simulink model "SmithPredictor"  (R2014a)
settings: Solver=ode45  StartTime=0.0  StopTime=200  RelTol=1e-3
libraries: simulink x2
settings Model: Creator=tri  LastModifiedBy=tri

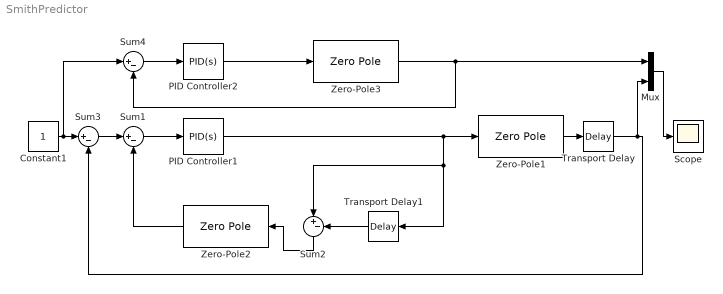
== system SmithPredictor ==
  Constant1 : Constant
  Mux : Mux  Inputs=2
  PID Controller1 : simulink/Continuous/PID Controller  Controller=PID  TimeDomain=Continuous-time  SampleTime=1  IntegratorMethod=Forward Euler  FilterMethod=Forward Euler  Form=Parallel  P=3  I=1/50  D=0  N=500  InitialConditionSource=internal  InitialConditionForIntegrator=0  InitialConditionForFilter=0  ExternalReset=none  LimitOutput=off  UpperSaturationLimit=inf  LowerSaturationLimit=-inf  LinearizeAsGain=on  AntiWindupMode=none  Kb=1  TrackingMode=off  Kt=1  PParamMin=[]  PParamMax=[]  IParamMin=[]  IParamMax=[]  DParamMin=[]  DParamMax=[]  NParamMin=[]  NParamMax=[]  KbParamMin=[]  KbParamMax=[]  KtParamMin=[]  KtParamMax=[]  POutMin=[]  POutMax=[]  IOutMin=[]  IOutMax=[]  DOutMin=[]  DOutMax=[]  NOutMin=[]  NOutMax=[]  KbOutMin=[]  KbOutMax=[]  KtOutMin=[]  KtOutMax=[]  IntegratorOutMin=[]  IntegratorOutMax=[]  FilterOutMin=[]  FilterOutMax=[]  SumOutMin=[]  SumOutMax=[]  SumI1OutMin=[]  SumI1OutMax=[]  SumI2OutMin=[]  SumI2OutMax=[]  SumI3OutMin=[]  SumI3OutMax=[]  SumDOutMin=[]  SumDOutMax=[]  SaturationOutMin=[]  SaturationOutMax=[]  IntegratorContinuousStateAttributes=''  IntegratorStateMustResolveToSignalObject=off  IntegratorRTWStateStorageClass=Auto  FilterContinuousStateAttributes=''  FilterStateMustResolveToSignalObject=off  FilterRTWStateStorageClass=Auto
  PID Controller2 : simulink/Continuous/PID Controller  Controller=PID  TimeDomain=Continuous-time  SampleTime=1  IntegratorMethod=Forward Euler  FilterMethod=Forward Euler  Form=Parallel  P=3  I=1/50  D=0  N=500  InitialConditionSource=internal  InitialConditionForIntegrator=0  InitialConditionForFilter=0  ExternalReset=none  LimitOutput=off  UpperSaturationLimit=inf  LowerSaturationLimit=-inf  LinearizeAsGain=on  AntiWindupMode=none  Kb=1  TrackingMode=off  Kt=1  PParamMin=[]  PParamMax=[]  IParamMin=[]  IParamMax=[]  DParamMin=[]  DParamMax=[]  NParamMin=[]  NParamMax=[]  KbParamMin=[]  KbParamMax=[]  KtParamMin=[]  KtParamMax=[]  POutMin=[]  POutMax=[]  IOutMin=[]  IOutMax=[]  DOutMin=[]  DOutMax=[]  NOutMin=[]  NOutMax=[]  KbOutMin=[]  KbOutMax=[]  KtOutMin=[]  KtOutMax=[]  IntegratorOutMin=[]  IntegratorOutMax=[]  FilterOutMin=[]  FilterOutMax=[]  SumOutMin=[]  SumOutMax=[]  SumI1OutMin=[]  SumI1OutMax=[]  SumI2OutMin=[]  SumI2OutMax=[]  SumI3OutMin=[]  SumI3OutMax=[]  SumDOutMin=[]  SumDOutMax=[]  SaturationOutMin=[]  SaturationOutMax=[]  IntegratorContinuousStateAttributes=''  IntegratorStateMustResolveToSignalObject=off  IntegratorRTWStateStorageClass=Auto  FilterContinuousStateAttributes=''  FilterStateMustResolveToSignalObject=off  FilterRTWStateStorageClass=Auto
  Scope : Scope
      settings: TimeRange=200  YMin=0  YMax=2
  Sum{1..4} (4 alike) : Sum  Inputs=|+-
  Transport Delay : TransportDelay  DelayTime=5
  Transport Delay1 : TransportDelay  DelayTime=5
  Zero-Pole1 : ZeroPole  Zeros=[]  Poles=[-0.1 -1/150 ]  Gain=2.5/1500
  Zero-Pole2 : ZeroPole  Zeros=[]  Poles=[-0.1 -1/150 ]  Gain=2.5/1500
  Zero-Pole3 : ZeroPole  Zeros=[]  Poles=[-0.1 -1/150 ]  Gain=2.5/1500
  wires:
  Sum1/1 -> PID Controller1/1
  Zero-Pole1/1 -> Transport Delay/1
  Zero-Pole2/1 -> Sum1/2
  Sum3/1 -> Sum1/1
  Constant1/1 -> Sum4/1, Sum3/1
  Sum2/1 -> Zero-Pole2/1
  Transport Delay1/1 -> Sum2/2
  PID Controller1/1 -> Zero-Pole1/1, Transport Delay1/1, Sum2/1
  Transport Delay/1 -> Mux/2, Sum3/2
  Sum4/1 -> PID Controller2/1
  PID Controller2/1 -> Zero-Pole3/1
  Zero-Pole3/1 -> Sum4/2, Mux/1
  Mux/1 -> Scope/1
